simulink model "modelPID"  (R2015b)
settings: Solver=VariableStepAuto  StartTime=0.0  StopTime=10.0  RelTol=1e-3
values from neighbouring files (symbols this model uses):
  Beff = 1/80    (= 0.0125)    [commande_robot.m]    (also in sf_loi_avant_RP.m; sf_retour_linearisant_RP.m)
  Jeff = Jm + r^2*m    [commande_robot.m]    (also in sf_loi_avant_RP.m = Jm+r^2*m; sf_retour_linearisant_RP.m = Jm+r^2*m)
  K = (Kd^2)/4    (= 2.25)    [commande_robot.m]
  Kd = 3    [commande_robot.m]
  Km_R = 0.3    [commande_robot.m]    (also in sf_loi_avant_RP.m; sf_retour_linearisant_RP.m)
  r = R(1)    [commande_robot.m]    (also in sf_loi_avant_RP.m; sf_retour_linearisant_RP.m)
  Ti = 20000    [commande_robot.m]
  Ti2 = 12    [commande_robot.m]
libraries: lib_robotRP x2, simulink x1, cstblocks x1
settings Model: Creator=chamand  LastModifiedBy=chamand

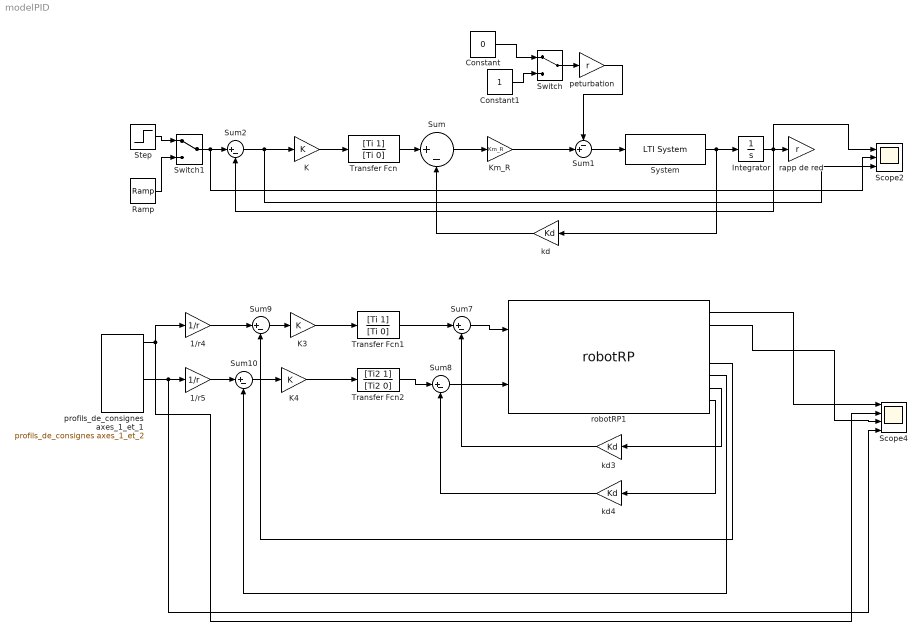
== system modelPID ==
  1/r4 : Gain  Gain=1/r
  1/r5 : Gain  Gain=1/r
  Constant : Constant  Value=0
  Constant1 : Constant
  Integrator : Integrator
  K : Gain  Gain=K
  K3 : Gain  Gain=K
  K4 : Gain  Gain=K
  "Km_R " : Gain  Gain=Km_R
  Ramp : simulink/Sources/Ramp  slope=1  start=0  X0=0
  Scope2 : Scope  NumInputPorts=3
  Scope4 : Scope  NumInputPorts=4
  Step : Step  Time=0  SampleTime=0
  Sum{,2,7..10} (6 alike) : Sum  Inputs=|+-
  Sum1 : Sum  Inputs=-+|
  Switch : ManualSwitch
  Switch1 : ManualSwitch
  System : cstblocks/LTI System  sys=tf(1,[Jeff Beff])  IC=[]
  Transfer Fcn : TransferFcn  Numerator=[Ti 1]  Denominator=[Ti 0]
  Transfer Fcn1 : TransferFcn  Numerator=[Ti 1]  Denominator=[Ti 0]
  Transfer Fcn2 : TransferFcn  Numerator=[Ti2 1]  Denominator=[Ti2 0]
  kd : Gain  Gain=Kd
  kd3 : Gain  Gain=Kd
  kd4 : Gain  Gain=Kd
  peturbation : Gain  Gain=r
  profils_de_consignes axes_1_et_1 : lib_robotRP/profils_de_consignes axes_1_et_2
  "rapp de red " : Gain  Gain=r
  robotRP1 : lib_robotRP/robotRP  vecteur_theta_dtheta_initial=[0 ; 1/2/r ; 0 ; 0]  m=15  gX=0  gY=-9.81  F1=0  F2=0  H1=0  H2=0  Km_sur_R=0.3  Jm=0.01  Beff=0.0125  r=1/200
  wires:
  Sum7/1 -> robotRP1/1
  robotRP1/7 -> kd3/1
  robotRP1/5 -> Sum9/2
  robotRP1/1 -> Scope4/1
  Sum9/1 -> K3/1
  robotRP1/2 -> Scope4/3
  robotRP1/8 -> kd4/1
  robotRP1/6 -> Sum10/2
  Sum10/1 -> K4/1
  Sum8/1 -> robotRP1/2
  profils_de_consignes axes_1_et_1/1 -> 1/r4/1, Scope4/2
  profils_de_consignes axes_1_et_1/4 -> Scope4/4, 1/r5/1
  1/r5/1 -> Sum10/1
  1/r4/1 -> Sum9/1
  Sum/1 -> "Km_R "/1
  System/1 -> kd/1, Integrator/1
  Constant/1 -> Switch/1
  Switch/1 -> peturbation/1
  "Km_R "/1 -> Sum1/2
  peturbation/1 -> Sum1/1
  Sum1/1 -> System/1
  Step/1 -> Switch1/1
  Ramp/1 -> Switch1/2
  Sum2/1 -> K/1, Scope2/3
  Switch1/1 -> Scope2/2, Sum2/1
  Constant1/1 -> Switch/2
  Integrator/1 -> Scope2/1, Sum2/2, "rapp de red "/1
  K/1 -> Transfer Fcn/1
  kd/1 -> Sum/2
  Transfer Fcn/1 -> Sum/1
  K3/1 -> Transfer Fcn1/1
  Transfer Fcn1/1 -> Sum7/1
  kd3/1 -> Sum7/2
  Transfer Fcn2/1 -> Sum8/1
  K4/1 -> Transfer Fcn2/1
  kd4/1 -> Sum8/2
